simulink model "Blending_Tank"  (R2015b)
settings: Solver=VariableStepAuto  StartTime=0.0  StopTime=20  RelTol=1e-3
settings Model: Creator=Emsnuelly  LastModifiedBy=Emsnuelly

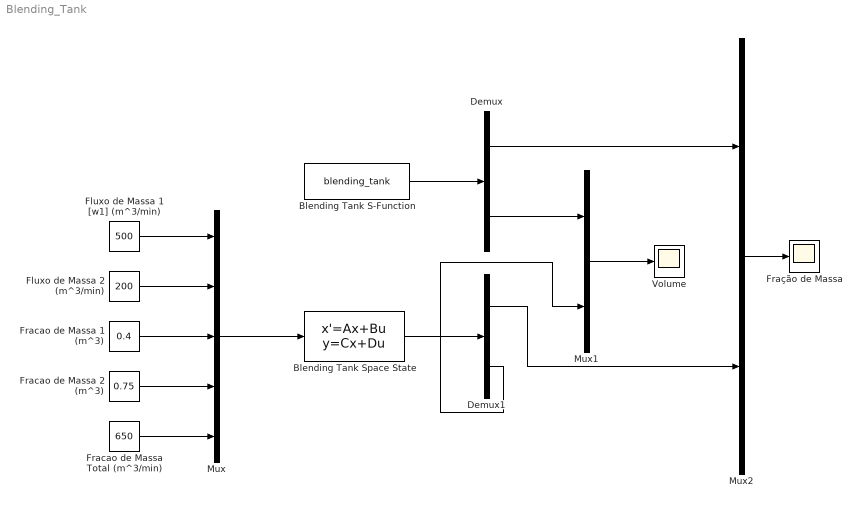
== system Blending_Tank ==
  Blending Tank S-Function : S-Function  FunctionName=blending_tank  Parameters=w1,w2,w,x1,x2,p  SFunctionDeploymentMode=off  EnableBusSupport=off  mask{w1=500, w2=200, w=650, x1=0.4, x2=0.75, p=900}
      mask prompts: w1 "Fluxo de Massa 1 [w1]  (m^3/min)"; w2 "Fluxo de Massa 2 [w2] (m^3/min)"; w "Fluxo de Massa Total [w] (m^3/min)"; x1 "Fração de Massa 1 [x1] (m^3)"; x2 "Fração de Massa 2 [x2](m^3)"; p "Densidade (p) (kg/m^3)"
  Blending Tank Space State : StateSpace  A=[-0.3703 0 ; 0 0]  B=[-0.0000529 0.00007936 0.2645 0.1058 0 ; 0.0011 0.0011 0 0 -0.0011]  C=[1 0 ; 0 1]  D=[0 0 0 0 0 ; 0 0 0 0 0]  X0=[0 2]
  Demux : Demux  Outputs=2
  Demux1 : Demux  Outputs=2
  Fluxo de Massa 1 [w1] (m^3/min) : Constant  Value=500
  Fluxo de Massa 2 (m^3/min) : Constant  Value=200
  Fracao de Massa 1 (m^3) : Constant  Value=0.4
  Fracao de Massa 2 (m^3) : Constant  Value=0.75
  Fracao de Massa Total (m^3/min) : Constant  Value=650
  Fração de Massa : Scope
  Mux : Mux  Inputs=5
  Mux1 : Mux  Inputs=2
  Mux2 : Mux  Inputs=2
  Volume : Scope
  wires:
  Blending Tank S-Function/1 -> Demux/1
  Mux/1 -> Blending Tank Space State/1
  Blending Tank Space State/1 -> Demux1/1
  Fluxo de Massa 1 [w1] (m^3/min)/1 -> Mux/1
  Mux1/1 -> Volume/1
  Mux2/1 -> Fração de Massa/1
  Fluxo de Massa 2 (m^3/min)/1 -> Mux/2
  Fracao de Massa 1 (m^3)/1 -> Mux/3
  Fracao de Massa Total (m^3/min)/1 -> Mux/5
  Fracao de Massa 2 (m^3)/1 -> Mux/4
  Demux/1 -> Mux2/1
  Demux/2 -> Mux1/1
  Demux1/1 -> Mux2/2
  Demux1/2 -> Mux1/2
